simulink library "ccmotor_lib"  (R2017a)
settings: Solver=VariableStepAuto  StartTime=0.0  StopTime=10.0  RelTol=1e-3
settings Model: Creator=jdam  LastModifiedBy=jdam

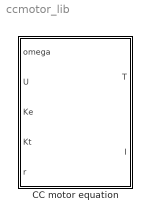
== system ccmotor_lib ==
  CC motor equation : Subsystem

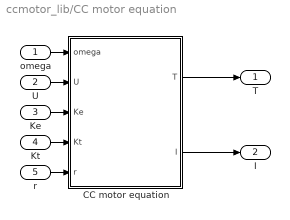
== system ccmotor_lib/CC motor equation ==
  omega : Inport
  U : Inport  Port=2
  Ke : Inport  Port=3
  Kt : Inport  Port=4
  r : Inport  Port=5
  CC motor equation : MATLAB Function  TreatAsAtomicUnit=on
  T : Outport
  I : Outport  Port=2
  wires:
  r/1 -> CC motor equation/5(r)
  Ke/1 -> CC motor equation/3(Ke)
  U/1 -> CC motor equation/2(U)
  Kt/1 -> CC motor equation/4(Kt)
  CC motor equation/1(T) -> T/1
  omega/1 -> CC motor equation/1(omega)
  CC motor equation/2(I) -> I/1

== matlab function ccmotor_lib/CC motor equation/CC motor equation ==
  data: omega input; T output; U input; Ke input; Kt input; r input; I output
function [T,I]= fcn(omega,U,Ke,Kt,r)
% torque
T = (U - Ke*omega)*Kt/r;
% current
I = T/Kt;
